simulink model "dspwpr"  (Simulink 6.0)
settings: Solver=FixedStepDiscrete  SolverMode=SingleTasking  StartTime=0.0  StopTime=1024  RelTol=1e-3
PreLoadFcn:
  | load dspwlets;
values from neighbouring files (symbols this model uses):
  ts = get_param(blk,'CompiledSampleTime')    [sdspwwvdisp.m]
undefined symbols (not defined in the file or in its folder): lod
libraries: dspmlti4 x6, dspsigops x3, dspsrcs4 x1
settings Model: Creator=don  LastModifiedBy=sconahan  ExtModeTrigMode=oneshot  ExtModeArmWhenConnect=off
settings DataIOCC: LimitDataPoints=off  SaveOutput=off  SaveTime=off  SignalLoggingName=sigsOut
settings OptimizationCC: BlockReduction=off  BooleanDataType=off  MultiInstanced=off
settings FormatCC: IgnoreBidirectionalLines=off
settings DebuggingCC: IntegerOverflowMsg=none
settings HardwareCC: TargetUnknown=on
settings CodeAppCC: FileBanners=off  CustomSymbols=off
settings GRTTargetCC: TargetFcnLib=iso_c_tmw.mat  IsERTTarget=off

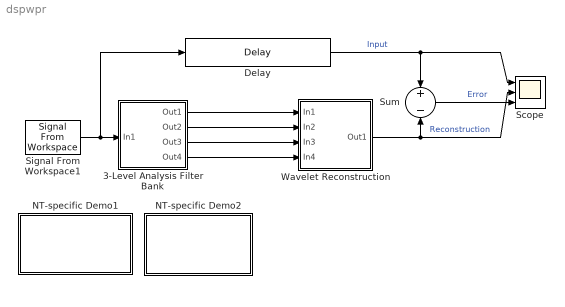
== system dspwpr ==
  3-Level Analysis Filter Bank : Subsystem
  Delay : dspsigops/Delay  dly_unit=Samples  delay=7*(length(lod)-1)  ic_detail=on  dif_ic_for_ch=off  dif_ic_for_dly=off  ic=0  reset_popup=None
  NT-specific Demo1 : Subsystem
      settings: OpenFcn=dspwprf
      mask Type: Frame-Based Demo
      mask Display: disp('Frame-Based\nDemo')
  NT-specific Demo2 : Subsystem
      settings: OpenFcn=dspwprfp
      mask Type: Fixed-Point Demo
      mask Display: disp('Fixed-Point\nDemo')
  Scope : Scope  NumInputPorts=3
      settings: TimeRange=1200  YMin=-10~-10~-10  YMax=10~10~10
  Signal From Workspace1 : dspsrcs4/Signal From Workspace  X=noisdopp  Ts=ts  nsamps=1  OutputAfterFinalValue=Setting to zero
  Sum : Sum  Inputs=+-  SaturateOnIntegerOverflow=on  InputSameDT=on
  Wavelet Reconstruction : Subsystem
  wires:
  Signal From Workspace1/1 -> 3-Level Analysis Filter Bank/1(In1), Delay/1
  Delay/1 -> Sum/1, Scope/1  "Input"
  Sum/1 -> Scope/3  "Error"
  3-Level Analysis Filter Bank/1(Out1) -> Wavelet Reconstruction/1(In1)
  3-Level Analysis Filter Bank/2(Out2) -> Wavelet Reconstruction/2(In2)
  3-Level Analysis Filter Bank/3(Out3) -> Wavelet Reconstruction/3(In3)
  3-Level Analysis Filter Bank/4(Out4) -> Wavelet Reconstruction/4(In4)
  Wavelet Reconstruction/1(Out1) -> Sum/2, Scope/2  "Reconstruction"

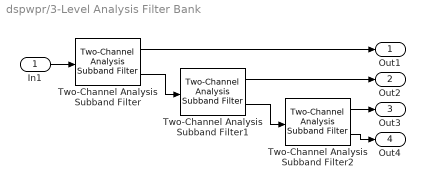
== system dspwpr/3-Level Analysis Filter Bank ==
  In1 : Inport
  Two-Channel Analysis Subband Filter : dspmlti4/Two-Channel Analysis Subband Filter  lpf=lod  hpf=hid  framing=Maintain input frame size  roundingMode=Floor  overflowMode=off
  Two-Channel Analysis Subband Filter1 : dspmlti4/Two-Channel Analysis Subband Filter  lpf=lod  hpf=hid  framing=Maintain input frame size  roundingMode=Floor  overflowMode=off
  Two-Channel Analysis Subband Filter2 : dspmlti4/Two-Channel Analysis Subband Filter  lpf=lod  hpf=hid  framing=Maintain input frame size  roundingMode=Floor  overflowMode=off
  Out1 : Outport
  Out2 : Outport  Port=2
  Out3 : Outport  Port=3
  Out4 : Outport  Port=4
  wires:
  Two-Channel Analysis Subband Filter2/2 -> Out4/1
  Two-Channel Analysis Subband Filter2/1 -> Out3/1
  Two-Channel Analysis Subband Filter1/1 -> Out2/1
  In1/1 -> Two-Channel Analysis Subband Filter/1
  Two-Channel Analysis Subband Filter/1 -> Out1/1
  Two-Channel Analysis Subband Filter1/2 -> Two-Channel Analysis Subband Filter2/1
  Two-Channel Analysis Subband Filter/2 -> Two-Channel Analysis Subband Filter1/1

== system dspwpr/NT-specific Demo1 ==

== system dspwpr/NT-specific Demo2 ==

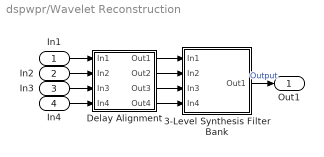
== system dspwpr/Wavelet Reconstruction ==
  In1 : Inport
  In2 : Inport  Port=2
  In3 : Inport  Port=3
  In4 : Inport  Port=4
  3-Level Synthesis Filter Bank : Subsystem
  Delay Alignment : Subsystem
  Out1 : Outport
  wires:
  Delay Alignment/1(Out1) -> 3-Level Synthesis Filter Bank/1(In1)
  Delay Alignment/2(Out2) -> 3-Level Synthesis Filter Bank/2(In2)
  Delay Alignment/3(Out3) -> 3-Level Synthesis Filter Bank/3(In3)
  Delay Alignment/4(Out4) -> 3-Level Synthesis Filter Bank/4(In4)
  In1/1 -> Delay Alignment/1(In1)
  In2/1 -> Delay Alignment/2(In2)
  3-Level Synthesis Filter Bank/1(Out1) -> Out1/1  "Output"
  In3/1 -> Delay Alignment/3(In3)
  In4/1 -> Delay Alignment/4(In4)

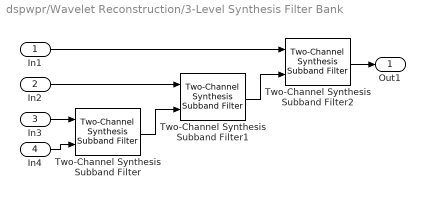
== system dspwpr/Wavelet Reconstruction/3-Level Synthesis Filter Bank ==
  In1 : Inport
  In2 : Inport  Port=2
  In3 : Inport  Port=3
  In4 : Inport  Port=4
  Two-Channel Synthesis Subband Filter : dspmlti4/Two-Channel Synthesis Subband Filter  lpf=lor  hpf=hir  framing=Maintain input frame size  roundingMode=Floor  overflowMode=off
  Two-Channel Synthesis Subband Filter1 : dspmlti4/Two-Channel Synthesis Subband Filter  lpf=lor  hpf=hir  framing=Maintain input frame size  roundingMode=Floor  overflowMode=off
  Two-Channel Synthesis Subband Filter2 : dspmlti4/Two-Channel Synthesis Subband Filter  lpf=lor  hpf=hir  framing=Maintain input frame size  roundingMode=Floor  overflowMode=off
  Out1 : Outport
  wires:
  In4/1 -> Two-Channel Synthesis Subband Filter/2
  In3/1 -> Two-Channel Synthesis Subband Filter/1
  In2/1 -> Two-Channel Synthesis Subband Filter1/1
  Two-Channel Synthesis Subband Filter2/1 -> Out1/1
  In1/1 -> Two-Channel Synthesis Subband Filter2/1
  Two-Channel Synthesis Subband Filter1/1 -> Two-Channel Synthesis Subband Filter2/2
  Two-Channel Synthesis Subband Filter/1 -> Two-Channel Synthesis Subband Filter1/2

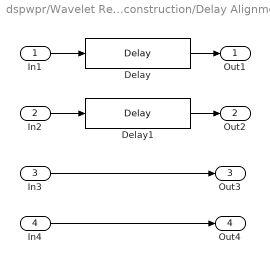
== system dspwpr/Wavelet Reconstruction/Delay Alignment ==
  In1 : Inport
  In2 : Inport  Port=2
  In3 : Inport  Port=3
  In4 : Inport  Port=4
  Delay : dspsigops/Delay  dly_unit=Samples  delay=3*(length(lod)-1)  ic_detail=on  dif_ic_for_ch=off  dif_ic_for_dly=off  ic=0  reset_popup=None
  Delay1 : dspsigops/Delay  dly_unit=Samples  delay=length(lod) - 1  ic_detail=on  dif_ic_for_ch=off  dif_ic_for_dly=off  ic=0  reset_popup=None
  Out1 : Outport
  Out2 : Outport  Port=2
  Out3 : Outport  Port=3
  Out4 : Outport  Port=4
  wires:
  In3/1 -> Out3/1
  In4/1 -> Out4/1
  In2/1 -> Delay1/1
  Delay1/1 -> Out2/1
  In1/1 -> Delay/1
  Delay/1 -> Out1/1
